simulink model "rtwdemo_export_functions"  (Simulink 7.6)
settings: Solver=FixedStepDiscrete  StartTime=0.0  StopTime=0.025  FixedStep=0.001  MaxStep=.0001  RelTol=1e-3
Description:
  | Exporting Function-Call Subsystems
CloseFcn:
  | rtwprivate ssgencode ModelCloseRequest case1_modified
settings Model: Creator=The MathWorks Inc.  ExtModeAutoUpdateStatusClock=off
settings MATStruct: SampleTime=0.001  Offset=0  Priority=[20.0]
settings DataIOCC: SaveOutput=off  SaveTime=off
settings OptimizationCC: InlineParams=on  InlineInvariantSignals=on  PassReuseOutputArgsAs=Individual arguments  StateBitsets=on  DataBitsets=on  UseTempVars=on  ZeroExternalMemoryAtStartup=off  ZeroInternalMemoryAtStartup=off  NoFixptDivByZeroProtection=on  EfficientFloat2IntCast=on  EfficientMapNaN2IntZero=off  OptimizeModelRefInitCode=on  LifeSpan=1  BufferReusableBoundary=off
settings DebuggingCC: SolverPrmCheckMsg=none  SigSpecEnsureSampleTimeMsg=none  BusObjectLabelMismatch=none  StrictBusMsg=ErrorOnBusTreatedAsVector
settings HardwareCC: ProdIntDivRoundTo=Zero  ProdEndianess=LittleEndian  ProdHWDeviceType=Generic->32-bit Embedded Processor  TargetIntDivRoundTo=Zero  TargetEndianess=LittleEndian  TargetHWDeviceType=Generic->32-bit Embedded Processor
settings SFSimCC: SimParseCustomCode=off
settings RTWCC: SystemTargetFile=ert.tlc  TemplateMakefile=ert_default_tmf  Description=Real-Time Workshop Embedded Coder (no auto configuration)  GenerateReport=on  RTWVerbose=off  ProcessScript=ert_make_rtw_hook  IncludeHyperlinkInReport=on  LaunchReport=on
settings CodeAppCC: ForceParamTrailComments=on  IgnoreCustomStorageClasses=off  IgnoreTestpoints=on  SimulinkDataObjDesc=on  CustomSymbolStrGlobalVar=rt$N$M  CustomSymbolStrType=$N$M  CustomSymbolStrFcn=$N$M$F  CustomSymbolStrMacro=$N$M  InsertBlockDesc=on
settings ERTTargetCC: TargetFcnLib=ansi_tfl_tmw.mat  MultiwordLength=2048  GenerateSampleERTMain=on  IncludeMdlTerminateFcn=off  SupportNonFinite=off  SupportComplex=off  PortableWordSizes=on  InlinedParameterPlacement=NonHierarchical  ERTCustomFileTemplate=example_file_process.tlc  ERTFilePackagingFormat=CompactWithDataFile  ConvertIfToSwitch=off

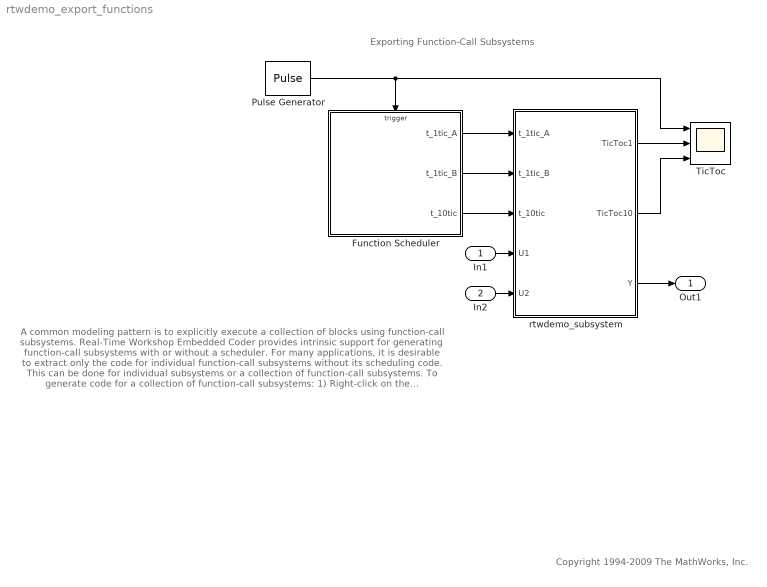
== system rtwdemo_export_functions ==
  note: Copyright 1994-2009 The MathWorks, Inc.
  note: Exporting Function-Call Subsystems
  note: A common modeling pattern is to explicitly execute a collection of blocks using function-call
      | subsystems. Real-Time Workshop Embedded Coder provides intrinsic support for generating
      | function-call subsystems with or without a scheduler.
      |
      | For many applications, it is desirable to extract only the code for individual function-call subsystems
      | without its scheduling code.  This can be done for individual subsystems or a collection of
      | function-call subsystems.
      |
      | To generate code for a collection of function-call subsystems:
      |
      | 1) Right-click on the 'rtwdemo_subsystem' subsystem and select Real-Time Workshop > Export Functions...
      | 2) Click the 'Build' button once the parameter dialog appears
  In1 : Inport  OutDataTypeStr=double  PortDimensions=1  SampleTime=0.001
  In2 : Inport  Port=2  OutDataTypeStr=double  PortDimensions=1  SampleTime=0.001
  Function Scheduler : Stateflow chart  TreatAsAtomicUnit=on
  Pulse Generator : DiscretePulseGenerator  SampleTime=.001
  TicToc : Scope  NumInputPorts=3
      settings: TimeRange=0.025  YMin=0~-1~-1  YMax=1~1~1
  rtwdemo_subsystem : Subsystem
  Out1 : Outport
  wires:
  Function Scheduler/1(t_1tic_A) -> rtwdemo_subsystem/1(t_1tic_A)
  Function Scheduler/2(t_1tic_B) -> rtwdemo_subsystem/2(t_1tic_B)
  Pulse Generator/1 -> Function Scheduler/Trigger, TicToc/1
  In1/1 -> rtwdemo_subsystem/4(U1)
  In2/1 -> rtwdemo_subsystem/5(U2)
  rtwdemo_subsystem/3(Y) -> Out1/1
  rtwdemo_subsystem/2(TicToc10) -> TicToc/3
  rtwdemo_subsystem/1(TicToc1) -> TicToc/2
  Function Scheduler/3(t_10tic) -> rtwdemo_subsystem/3(t_10tic)

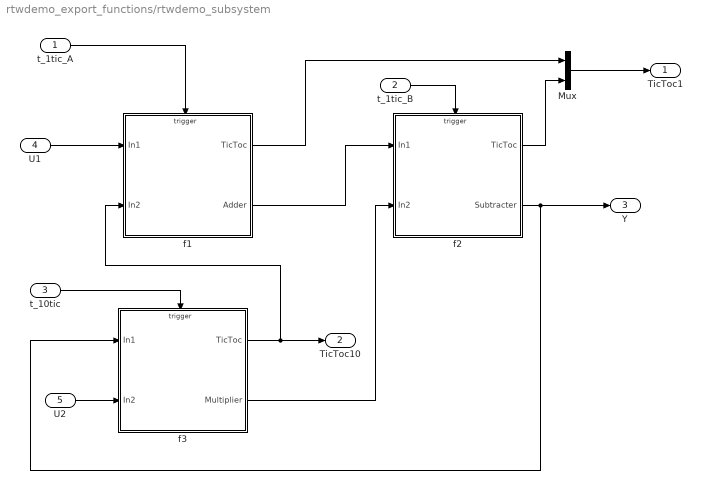
== system rtwdemo_export_functions/rtwdemo_subsystem ==
  t_1tic_A : Inport
  t_1tic_B : Inport  Port=2
  t_10tic : Inport  Port=3
  U1 : Inport  Port=4
  U2 : Inport  Port=5
  Mux : Mux  Inputs=2
  f1 : Subsystem  TreatAsAtomicUnit=on  RTWFcnName=foo
  f2 : Subsystem  TreatAsAtomicUnit=on  RTWFcnName=foo
  f3 : Subsystem  TreatAsAtomicUnit=on  RTWFcnName=foo
  TicToc1 : Outport
  TicToc10 : Outport  Port=2
  Y : Outport  Port=3
  wires:
  t_10tic/1 -> f3/Trigger
  U2/1 -> f3/2(In2)
  f2/2(Subtracter) -> Y/1, f3/1(In1)
  f1/2(Adder) -> f2/1(In1)
  f3/2(Multiplier) -> f2/2(In2)
  t_1tic_A/1 -> f1/Trigger
  f3/1(TicToc) -> f1/2(In2), TicToc10/1
  f2/1(TicToc) -> Mux/2
  Mux/1 -> TicToc1/1
  f1/1(TicToc) -> Mux/1
  t_1tic_B/1 -> f2/Trigger
  U1/1 -> f1/1(In1)

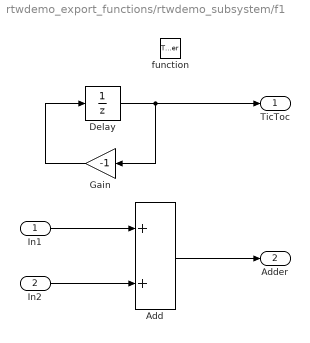
== system rtwdemo_export_functions/rtwdemo_subsystem/f1 ==
  In1 : Inport
  In2 : Inport  Port=2
  function : TriggerPort  TriggerType=function-call
  Add : Sum
  Delay : UnitDelay  X0=1  SampleTime=-1
  Gain : Gain  Gain=-1  OutDataTypeStr=fixdt(1,8,0)
  TicToc : Outport  InitialOutput=0
  Adder : Outport  Port=2  InitialOutput=0
  wires:
  Add/1 -> Adder/1
  Gain/1 -> Delay/1
  Delay/1 -> TicToc/1, Gain/1
  In1/1 -> Add/1
  In2/1 -> Add/2

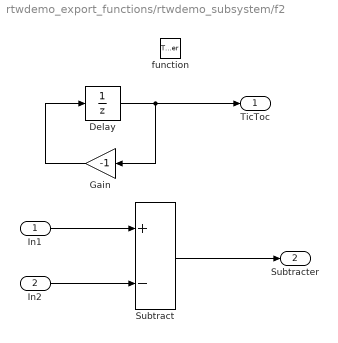
== system rtwdemo_export_functions/rtwdemo_subsystem/f2 ==
  In1 : Inport
  In2 : Inport  Port=2
  function : TriggerPort  TriggerType=function-call
  Delay : UnitDelay  X0=1  SampleTime=-1
  Gain : Gain  Gain=-1  OutDataTypeStr=fixdt(1,8,0)
  Subtract : Sum  Inputs=+-
  TicToc : Outport  InitialOutput=0
  Subtracter : Outport  Port=2  InitialOutput=0
  wires:
  In2/1 -> Subtract/2
  In1/1 -> Subtract/1
  Delay/1 -> Gain/1, TicToc/1
  Gain/1 -> Delay/1
  Subtract/1 -> Subtracter/1

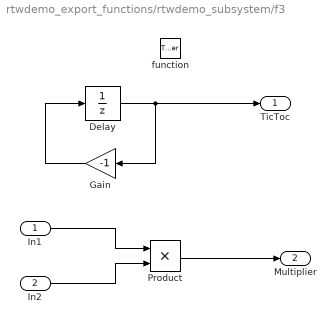
== system rtwdemo_export_functions/rtwdemo_subsystem/f3 ==
  In1 : Inport
  In2 : Inport  Port=2
  function : TriggerPort  TriggerType=function-call
  Delay : UnitDelay  X0=1  SampleTime=-1
  Gain : Gain  Gain=-1  OutDataTypeStr=fixdt(1,8,0)
  Product : Product  Inputs=**  OutDataTypeStr=Inherit: Same as first input
  TicToc : Outport  InitialOutput=0
  Multiplier : Outport  Port=2  InitialOutput=0
  wires:
  In2/1 -> Product/2
  In1/1 -> Product/1
  Delay/1 -> Gain/1, TicToc/1
  Gain/1 -> Delay/1
  Product/1 -> Multiplier/1

== stateflow chart Function Scheduler ==
  settings: executeAtInitialization=1
  state OneTic [parallel]
    on every(1,tic):
    t_1tic_B; t_1tic_A;
    settings: executionOrder=1
  state TenTic [parallel]
    on every(10,tic): t_10tic;
    settings: executionOrder=2
  events: tic input EITHER_EDGE_EVENT; t_1tic_A output FUNCTION_CALL_EVENT; t_1tic_B output FUNCTION_CALL_EVENT; t_10tic output FUNCTION_CALL_EVENT
